simulink model "spindle_mileusnic"  (Simulink 7.0)
settings: Solver=ode23s  StartTime=0.0  StopTime=3  RelTol=1e-3
values from neighbouring files (symbols this model uses):
  a = [0.3; 0.3; 0.3]    [SetSpindleConstants.m]    (also in createRamp.m = velocity / tacc)
  beta0 = [0.0605; 0.0822; 0.0822]    [SetSpindleConstants.m]
  beta1 = [0.2592; nan; nan]    [SetSpindleConstants.m]
  beta2 = [nan; -0.0460; -0.0690]    [SetSpindleConstants.m]
  Cl = [1; 1; 1]    [SetSpindleConstants.m]
  Cs = [0.42; 0.42; 0.42]    [SetSpindleConstants.m]
  freq = [60; 60; 90]    [SetSpindleConstants.m]
  Gamma1 = [0.0289; nan; nan]    [SetSpindleConstants.m]
  Gamma2 = [nan; 0.0636; 0.0954]    [SetSpindleConstants.m]
  Gprim = [20000; 10000; 10000]    [SetSpindleConstants.m]
  Gsec = [nan; 7250; 7250]    [SetSpindleConstants.m]
  Kpr = [0.15; 0.15; 0.15]    [SetSpindleConstants.m]
  Ksr = [10.4549; 10.4649; 10.4649]    [SetSpindleConstants.m]
  L0pr = [0.76; 0.76; 0.76]    [SetSpindleConstants.m]
  L0sr = [0.04; 0.04; 0.04]    [SetSpindleConstants.m]
  Lnpr = [nan; 0.89; 0.89]    [SetSpindleConstants.m]
  Lnsr = [0.0423; 0.0423; 0.0423]    [SetSpindleConstants.m]
  Lsec = [nan; 0.04; 0.04]    [SetSpindleConstants.m]
  M = M/100    [SetSpindleConstants.m]
  p = [2; 2; 2]    [SetSpindleConstants.m]
  R = [0.46; 0.46; 0.46]    [SetSpindleConstants.m]
  S = (E >= TH)    [RampModel.m]    (also in SetSpindleConstants.m = 0.156; step3_plotResults.m = out{velIdx,ampIdx}.nrn.Sdetail)
  tau = [0.0149; 0.205; nan]    [SetSpindleConstants.m]
  X = [nan; 0.7; 0.7]    [SetSpindleConstants.m]
settings Model: Creator=Schuurmans  LastModifiedBy=jschuurmans1
settings DebuggingCC: SaveWithParameterizedLinksMsg=none  SignalResolutionControl=TryResolveAllWithWarning  SolverPrmCheckMsg=none
settings GRTTargetCC: TargetFcnLib=ansi_tfl_tmw.mat

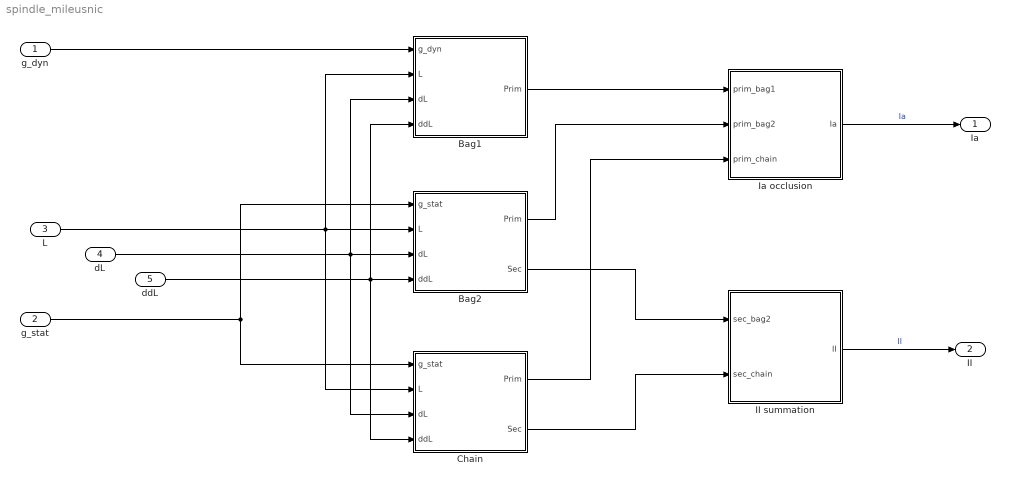
== system spindle_mileusnic ==
  g_dyn : Inport  OutDataType=sfix(16)  OutScaling=2^0
  g_stat : Inport  Port=2  OutDataType=sfix(16)  OutScaling=2^0
  L : Inport  Port=3  OutDataType=sfix(16)  OutScaling=2^0  Interpolate=off
  dL : Inport  Port=4  OutDataType=sfix(16)  OutScaling=2^0  Interpolate=off
  ddL : Inport  Port=5  OutDataType=sfix(16)  OutScaling=2^0  Interpolate=off
  Bag1 : Subsystem
  Bag2 : Subsystem
  Chain : Subsystem
  II summation : Subsystem
  Ia occlusion : Subsystem
  Ia : Outport  OutDataType=sfix(16)  OutScaling=2^0
  II : Outport  Port=2  OutDataType=sfix(16)  OutScaling=2^0
  wires:
  L/1 -> Bag2/2(L), Chain/2(L), Bag1/2(L)
  dL/1 -> Bag2/3(dL), Bag1/3(dL), Chain/3(dL)
  ddL/1 -> Bag2/4(ddL), Bag1/4(ddL), Chain/4(ddL)
  g_dyn/1 -> Bag1/1(g_dyn)
  g_stat/1 -> Bag2/1(g_stat), Chain/1(g_stat)
  Bag1/1(Prim) -> Ia occlusion/1(prim_bag1)
  Bag2/1(Prim) -> Ia occlusion/2(prim_bag2)
  Chain/1(Prim) -> Ia occlusion/3(prim_chain)
  Bag2/2(Sec) -> II summation/1(sec_bag2)
  Chain/2(Sec) -> II summation/2(sec_chain)
  II summation/1(II) -> II/1  "II"
  Ia occlusion/1(Ia) -> Ia/1  "Ia"

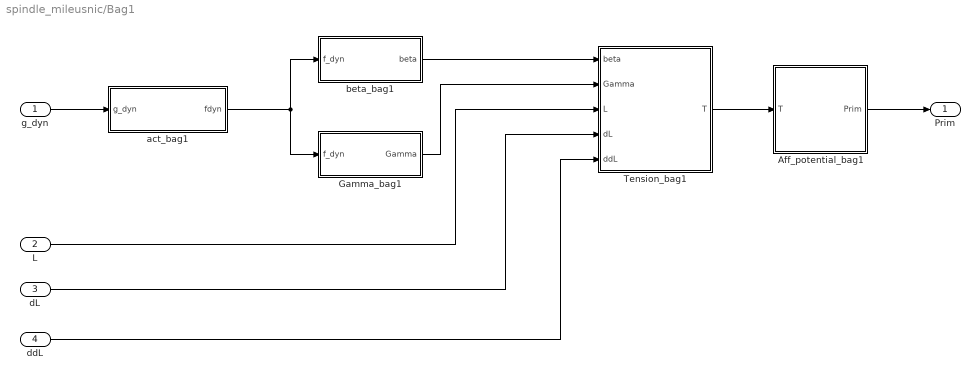
== system spindle_mileusnic/Bag1 ==
  g_dyn : Inport  OutDataType=sfix(16)  OutScaling=2^0
  L : Inport  Port=2  OutDataType=sfix(16)  OutScaling=2^0
  dL : Inport  Port=3  OutDataType=sfix(16)  OutScaling=2^0
  ddL : Inport  Port=4  OutDataType=sfix(16)  OutScaling=2^0
  Aff_potential_bag1 : Subsystem
  Gamma_bag1 : Subsystem
  Tension_bag1 : Subsystem
  act_bag1 : Subsystem
  beta_bag1 : Subsystem
  Prim : Outport  OutDataType=sfix(16)  OutScaling=2^0
  wires:
  act_bag1/1(fdyn) -> beta_bag1/1(f_dyn), Gamma_bag1/1(f_dyn)
  Gamma_bag1/1(Gamma) -> Tension_bag1/2(Gamma)
  Tension_bag1/1(T) -> Aff_potential_bag1/1(T)
  beta_bag1/1(beta) -> Tension_bag1/1(beta)
  g_dyn/1 -> act_bag1/1(g_dyn)
  L/1 -> Tension_bag1/3(L)
  dL/1 -> Tension_bag1/4(dL)
  ddL/1 -> Tension_bag1/5(ddL)
  Aff_potential_bag1/1(Prim) -> Prim/1

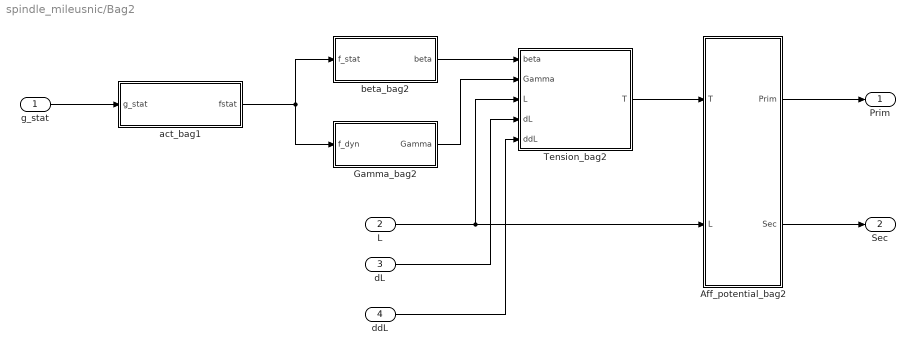
== system spindle_mileusnic/Bag2 ==
  g_stat : Inport  OutDataType=sfix(16)  OutScaling=2^0
  L : Inport  Port=2  OutDataType=sfix(16)  OutScaling=2^0
  dL : Inport  Port=3  OutDataType=sfix(16)  OutScaling=2^0
  ddL : Inport  Port=4  OutDataType=sfix(16)  OutScaling=2^0
  Aff_potential_bag2 : Subsystem
  Gamma_bag2 : Subsystem
  Tension_bag2 : Subsystem
  act_bag1 : Subsystem
  beta_bag2 : Subsystem
  Prim : Outport  OutDataType=sfix(16)  OutScaling=2^0
  Sec : Outport  Port=2  OutDataType=sfix(16)  OutScaling=2^0
  wires:
  g_stat/1 -> act_bag1/1(g_stat)
  beta_bag2/1(beta) -> Tension_bag2/1(beta)
  Gamma_bag2/1(Gamma) -> Tension_bag2/2(Gamma)
  act_bag1/1(fstat) -> beta_bag2/1(f_stat), Gamma_bag2/1(f_dyn)
  L/1 -> Tension_bag2/3(L), Aff_potential_bag2/2(L)
  dL/1 -> Tension_bag2/4(dL)
  ddL/1 -> Tension_bag2/5(ddL)
  Aff_potential_bag2/1(Prim) -> Prim/1
  Aff_potential_bag2/2(Sec) -> Sec/1
  Tension_bag2/1(T) -> Aff_potential_bag2/1(T)

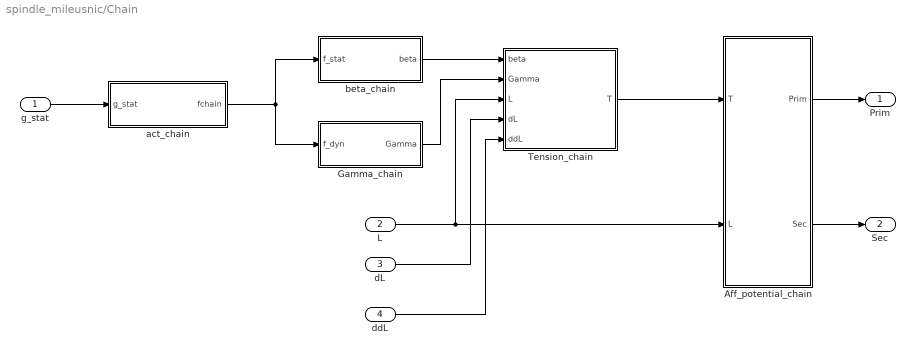
== system spindle_mileusnic/Chain ==
  g_stat : Inport  OutDataType=sfix(16)  OutScaling=2^0
  L : Inport  Port=2  OutDataType=sfix(16)  OutScaling=2^0
  dL : Inport  Port=3  OutDataType=sfix(16)  OutScaling=2^0
  ddL : Inport  Port=4  OutDataType=sfix(16)  OutScaling=2^0
  Aff_potential_chain : Subsystem
  Gamma_chain : Subsystem
  Tension_chain : Subsystem
  act_chain : Subsystem
  beta_chain : Subsystem
  Prim : Outport  OutDataType=sfix(16)  OutScaling=2^0
  Sec : Outport  Port=2  OutDataType=sfix(16)  OutScaling=2^0
  wires:
  beta_chain/1(beta) -> Tension_chain/1(beta)
  Gamma_chain/1(Gamma) -> Tension_chain/2(Gamma)
  act_chain/1(fchain) -> beta_chain/1(f_stat), Gamma_chain/1(f_dyn)
  g_stat/1 -> act_chain/1(g_stat)
  L/1 -> Tension_chain/3(L), Aff_potential_chain/2(L)
  dL/1 -> Tension_chain/4(dL)
  ddL/1 -> Tension_chain/5(ddL)
  Tension_chain/1(T) -> Aff_potential_chain/1(T)
  Aff_potential_chain/2(Sec) -> Sec/1
  Aff_potential_chain/1(Prim) -> Prim/1

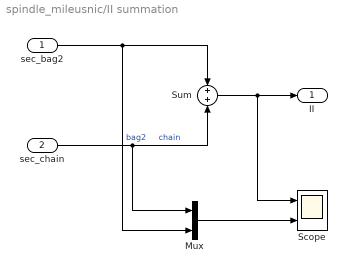
== system spindle_mileusnic/II summation ==
  sec_bag2 : Inport  OutDataType=sfix(16)  OutScaling=2^0
  sec_chain : Inport  Port=2  OutDataType=sfix(16)  OutScaling=2^0
  Mux : Mux  Inputs=2
  Scope : Scope  NumInputPorts=2
      settings: TickLabels=on  TimeRange=0.006999999999999673  YMin=0.00580385~-5  YMax=0.00580415~5  SaveName=ScopeData7
  Sum : Sum  OutDataType=sfix(16)  OutScaling=2^0
  II : Outport  OutDataType=sfix(16)  OutScaling=2^0
  wires:
  sec_bag2/1 -> Mux/2, Sum/1  "bag2"
  sec_chain/1 -> Sum/2, Mux/1  "chain"
  Sum/1 -> II/1, Scope/1
  Mux/1 -> Scope/2

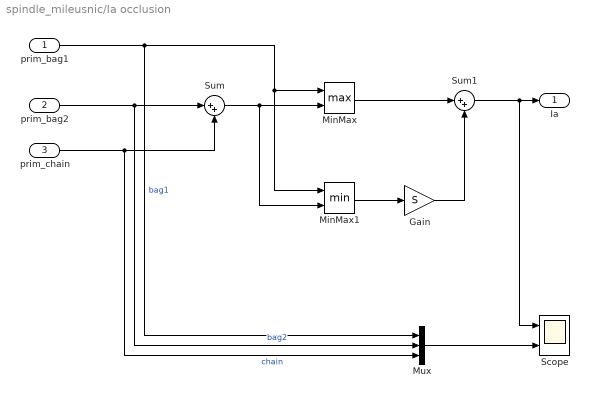
== system spindle_mileusnic/Ia occlusion ==
  prim_bag1 : Inport  OutDataType=sfix(16)  OutScaling=2^0
  prim_bag2 : Inport  Port=2  OutDataType=sfix(16)  OutScaling=2^0
  prim_chain : Inport  Port=3  OutDataType=sfix(16)  OutScaling=2^0
  Gain : Gain  Gain=S  ParameterDataType=sfix(16)  ParameterScaling=2^0  OutDataType=sfix(16)  OutScaling=2^0
  MinMax : MinMax  Function=max  Inputs=2  OutDataType=sfix(16)  OutScaling=2^0
  MinMax1 : MinMax  Inputs=2  OutDataType=sfix(16)  OutScaling=2^0
  Mux : Mux  Inputs=3
  Scope : Scope  NumInputPorts=2
      settings: TickLabels=on  TimeRange=0.006999999999999673  YMin=0.00580385~-5  YMax=0.00580415~5  SaveName=ScopeData5
  Sum : Sum  Inputs=|++  OutDataType=sfix(16)  OutScaling=2^0
  Sum1 : Sum  Inputs=|++  OutDataType=sfix(16)  OutScaling=2^0
  Ia : Outport  OutDataType=sfix(16)  OutScaling=2^0
  wires:
  prim_bag2/1 -> Sum/1, Mux/2  "bag2"
  prim_chain/1 -> Sum/2, Mux/3  "chain"
  prim_bag1/1 -> MinMax/1, MinMax1/1, Mux/1  "bag1"
  Sum/1 -> MinMax/2, MinMax1/2
  MinMax/1 -> Sum1/1
  MinMax1/1 -> Gain/1
  Gain/1 -> Sum1/2
  Sum1/1 -> Ia/1, Scope/1
  Mux/1 -> Scope/2

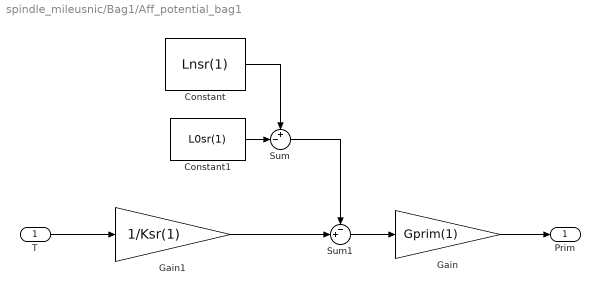
== system spindle_mileusnic/Bag1/Aff_potential_bag1 ==
  T : Inport  OutDataType=sfix(16)  OutScaling=2^0
  Constant : Constant  Value=Lnsr(1)  OutDataType=sfix(16)  OutScaling=2^0
  Constant1 : Constant  Value=L0sr(1)  OutDataType=sfix(16)  OutScaling=2^0
  Gain : Gain  Gain=Gprim(1)  ParameterDataType=sfix(16)  ParameterScaling=2^0  OutDataType=sfix(16)  OutScaling=2^0
  Gain1 : Gain  Gain=1/Ksr(1)  ParameterDataType=sfix(16)  ParameterScaling=2^0  OutDataType=sfix(16)  OutScaling=2^0
  Sum : Sum  Inputs=+-|  OutDataType=sfix(16)  OutScaling=2^0
  Sum1 : Sum  Inputs=-+|  OutDataType=sfix(16)  OutScaling=2^0
  Prim : Outport  OutDataType=sfix(16)  OutScaling=2^0
  wires:
  T/1 -> Gain1/1
  Constant1/1 -> Sum/2
  Constant/1 -> Sum/1
  Gain1/1 -> Sum1/2
  Sum/1 -> Sum1/1
  Sum1/1 -> Gain/1
  Gain/1 -> Prim/1

== system spindle_mileusnic/Bag1/Gamma_bag1 ==
  f_dyn : Inport  OutDataType=sfix(16)  OutScaling=2^0
  Gain : Gain  Gain=Gamma1(1)  ParameterDataType=sfix(16)  ParameterScaling=2^0  OutDataType=sfix(16)  OutScaling=2^0
  Gamma : Outport  OutDataType=sfix(16)  OutScaling=2^0
  wires:
  f_dyn/1 -> Gain/1
  Gain/1 -> Gamma/1

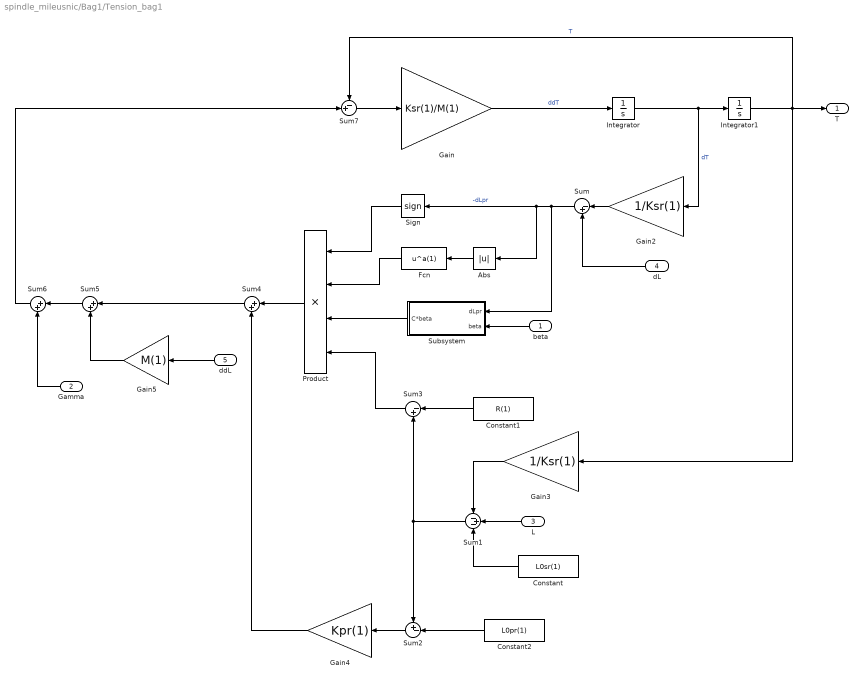
== system spindle_mileusnic/Bag1/Tension_bag1 ==
  beta : Inport  Orientation=left  OutDataType=sfix(16)  OutScaling=2^0
  Gamma : Inport  Orientation=left  Port=2  OutDataType=sfix(16)  OutScaling=2^0
  L : Inport  Orientation=left  Port=3  OutDataType=sfix(16)  OutScaling=2^0
  dL : Inport  Orientation=left  Port=4  OutDataType=sfix(16)  OutScaling=2^0
  ddL : Inport  Orientation=left  Port=5  OutDataType=sfix(16)  OutScaling=2^0
  Abs : Abs  Orientation=left  ZeroCross=off
  Constant : Constant  Orientation=left  Value=L0sr(1)  OutDataType=sfix(16)  OutScaling=2^0
  Constant1 : Constant  Orientation=left  Value=R(1)  OutDataType=sfix(16)  OutScaling=2^0
  Constant2 : Constant  Orientation=left  Value=L0pr(1)  OutDataType=sfix(16)  OutScaling=2^0
  Fcn : Fcn  Orientation=left  Expr=u^a(1)
  Gain : Gain  Gain=Ksr(1)/M(1)  ParameterDataType=sfix(16)  ParameterScaling=2^0  OutDataType=sfix(16)  OutScaling=2^0
  Gain2 : Gain  Orientation=left  Gain=1/Ksr(1)  ParameterDataType=sfix(16)  ParameterScaling=2^0  OutDataType=sfix(16)  OutScaling=2^0
  Gain3 : Gain  Orientation=left  Gain=1/Ksr(1)  ParameterDataType=sfix(16)  ParameterScaling=2^0  OutDataType=sfix(16)  OutScaling=2^0
  Gain4 : Gain  Orientation=left  Gain=Kpr(1)  ParameterDataType=sfix(16)  ParameterScaling=2^0  OutDataType=sfix(16)  OutScaling=2^0
  Gain5 : Gain  Orientation=left  Gain=M(1)  ParameterDataType=sfix(16)  ParameterScaling=2^0  OutDataType=sfix(16)  OutScaling=2^0
  Integrator : Integrator
  Integrator1 : Integrator
  Product : Product  Orientation=left  Inputs=4  OutDataType=sfix(16)  OutScaling=2^0  RndMeth=Zero
  Sign : Signum  Orientation=left  ZeroCross=off
  Subsystem : Subsystem  Orientation=left
  Sum : Sum  Orientation=left  Inputs=|-+  OutDataType=sfix(16)  OutScaling=2^0
  Sum1 : Sum  Orientation=left  Inputs=-+-  OutDataType=sfix(16)  OutScaling=2^0
  Sum2 : Sum  Orientation=left  Inputs=+-|  OutDataType=sfix(16)  OutScaling=2^0
  Sum3 : Sum  Orientation=left  Inputs=|-+  OutDataType=sfix(16)  OutScaling=2^0
  Sum4 : Sum  Orientation=left  Inputs=|++  OutDataType=sfix(16)  OutScaling=2^0
  Sum5 : Sum  Orientation=left  Inputs=|++  OutDataType=sfix(16)  OutScaling=2^0
  Sum6 : Sum  Orientation=left  Inputs=|++  OutDataType=sfix(16)  OutScaling=2^0
  Sum7 : Sum  Inputs=-+|  OutDataType=sfix(16)  OutScaling=2^0
  T : Outport  OutDataType=sfix(16)  OutScaling=2^0
  wires:
  Integrator/1 -> Integrator1/1, Gain2/1  "dT"
  Integrator1/1 -> Gain3/1, Sum7/1, T/1  "T"
  Gain/1 -> Integrator/1  "ddT"
  dL/1 -> Sum/2
  Gain2/1 -> Sum/1
  Sum/1 -> Sign/1, Abs/1, Subsystem/1(dLpr)  "-dLpr"
  Abs/1 -> Fcn/1
  Sign/1 -> Product/1
  Fcn/1 -> Product/2
  Sum3/1 -> Product/4
  L/1 -> Sum1/2
  Gain3/1 -> Sum1/1
  Constant/1 -> Sum1/3
  Sum1/1 -> Sum3/2, Sum2/1
  Constant1/1 -> Sum3/1
  Constant2/1 -> Sum2/2
  Sum2/1 -> Gain4/1
  ddL/1 -> Gain5/1
  Product/1 -> Sum4/1
  Gain4/1 -> Sum4/2
  Sum4/1 -> Sum5/1
  Gain5/1 -> Sum5/2
  Sum5/1 -> Sum6/1
  Gamma/1 -> Sum6/2
  Sum6/1 -> Sum7/2
  Sum7/1 -> Gain/1
  beta/1 -> Subsystem/2(beta)
  Subsystem/1(C*beta) -> Product/3

== system spindle_mileusnic/Bag1/act_bag1 ==
  g_dyn : Inport  OutDataType=sfix(16)  OutScaling=2^0
  Fcn : Fcn  Expr=u^p(1) / (u^p(1) + freq(1)^p(1))
  Gain : Gain  Gain=1/tau(1)  ParameterDataType=sfix(16)  ParameterScaling=2^0  OutDataType=sfix(16)  OutScaling=2^0
  Integrator : Integrator
  Sum : Sum  Inputs=|+-  OutDataType=sfix(16)  OutScaling=2^0
  fdyn : Outport  OutDataType=sfix(16)  OutScaling=2^0
  wires:
  Integrator/1 -> Sum/2, fdyn/1
  g_dyn/1 -> Fcn/1
  Fcn/1 -> Sum/1
  Gain/1 -> Integrator/1
  Sum/1 -> Gain/1

== system spindle_mileusnic/Bag1/beta_bag1 ==
  f_dyn : Inport  OutDataType=sfix(16)  OutScaling=2^0
  Gain : Gain  Gain=beta1(1)  ParameterDataType=sfix(16)  ParameterScaling=2^0  OutDataType=sfix(16)  OutScaling=2^0
  Sum : Sum  Inputs=|++  OutDataType=sfix(16)  OutScaling=2^0
  beta0 : Constant  Value=beta0(1)  OutDataType=sfix(16)  OutScaling=2^0
  beta : Outport  OutDataType=sfix(16)  OutScaling=2^0
  wires:
  f_dyn/1 -> Gain/1
  Gain/1 -> Sum/1
  beta0/1 -> Sum/2
  Sum/1 -> beta/1

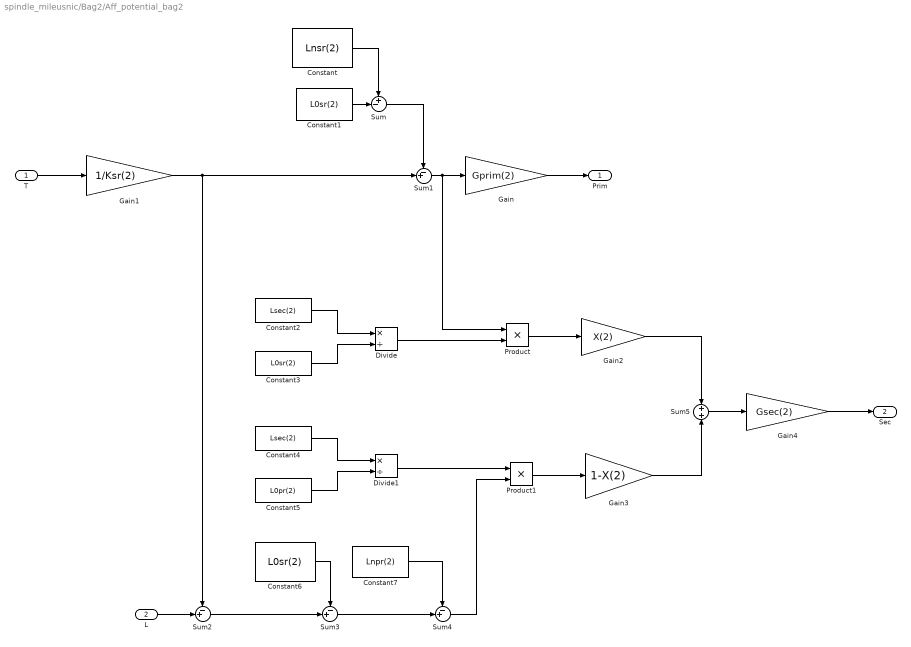
== system spindle_mileusnic/Bag2/Aff_potential_bag2 ==
  T : Inport  OutDataType=sfix(16)  OutScaling=2^0
  L : Inport  Port=2  OutDataType=sfix(16)  OutScaling=2^0
  Constant : Constant  Value=Lnsr(2)  OutDataType=sfix(16)  OutScaling=2^0
  Constant1 : Constant  Value=L0sr(2)  OutDataType=sfix(16)  OutScaling=2^0
  Constant2 : Constant  Value=Lsec(2)  OutDataType=sfix(16)  OutScaling=2^0
  Constant3 : Constant  Value=L0sr(2)  OutDataType=sfix(16)  OutScaling=2^0
  Constant4 : Constant  Value=Lsec(2)  OutDataType=sfix(16)  OutScaling=2^0
  Constant5 : Constant  Value=L0pr(2)  OutDataType=sfix(16)  OutScaling=2^0
  Constant6 : Constant  Value=L0sr(2)  OutDataType=sfix(16)  OutScaling=2^0
  Constant7 : Constant  Value=Lnpr(2)  OutDataType=sfix(16)  OutScaling=2^0
  Divide : Product  Inputs=*/  OutDataType=sfix(16)  OutScaling=2^-10
  Divide1 : Product  Inputs=*/  OutDataType=sfix(16)  OutScaling=2^-10
  Gain : Gain  Gain=Gprim(2)  ParameterDataType=sfix(16)  ParameterScaling=2^0  OutDataType=sfix(16)  OutScaling=2^0
  Gain1 : Gain  Gain=1/Ksr(2)  ParameterDataType=sfix(16)  ParameterScaling=2^0  OutDataType=sfix(16)  OutScaling=2^0
  Gain2 : Gain  Gain=X(2)  ParameterDataType=sfix(16)  ParameterScaling=2^0  OutDataType=sfix(16)  OutScaling=2^0
  Gain3 : Gain  Gain=1-X(2)  ParameterDataType=sfix(16)  ParameterScaling=2^0  OutDataType=sfix(16)  OutScaling=2^0
  Gain4 : Gain  Gain=Gsec(2)  ParameterDataType=sfix(16)  ParameterScaling=2^0  OutDataType=sfix(16)  OutScaling=2^0
  Product : Product  OutDataType=sfix(16)  OutScaling=2^0  RndMeth=Zero
  Product1 : Product  OutDataType=sfix(16)  OutScaling=2^0  RndMeth=Zero
  Sum : Sum  Inputs=+-|  OutDataType=sfix(16)  OutScaling=2^0
  Sum{1..4} (4 alike) : Sum  Inputs=-+|  OutDataType=sfix(16)  OutScaling=2^0
  Sum5 : Sum  Inputs=+|+  OutDataType=sfix(16)  OutScaling=2^0
  Prim : Outport  OutDataType=sfix(16)  OutScaling=2^0
  Sec : Outport  Port=2  OutDataType=sfix(16)  OutScaling=2^0
  wires:
  T/1 -> Gain1/1
  Constant1/1 -> Sum/2
  Constant/1 -> Sum/1
  Gain1/1 -> Sum1/2, Sum2/1
  Sum/1 -> Sum1/1
  Sum1/1 -> Gain/1, Product/1
  Gain/1 -> Prim/1
  Constant2/1 -> Divide/1
  Constant3/1 -> Divide/2
  Divide/1 -> Product/2
  Product/1 -> Gain2/1
  Constant4/1 -> Divide1/1
  Constant5/1 -> Divide1/2
  L/1 -> Sum2/2
  Sum2/1 -> Sum3/2
  Constant6/1 -> Sum3/1
  Sum3/1 -> Sum4/2
  Constant7/1 -> Sum4/1
  Divide1/1 -> Product1/1
  Sum4/1 -> Product1/2
  Product1/1 -> Gain3/1
  Gain2/1 -> Sum5/1
  Gain3/1 -> Sum5/2
  Sum5/1 -> Gain4/1
  Gain4/1 -> Sec/1

== system spindle_mileusnic/Bag2/Gamma_bag2 ==
  f_dyn : Inport  OutDataType=sfix(16)  OutScaling=2^0
  Gain : Gain  Gain=Gamma2(2)  ParameterDataType=sfix(16)  ParameterScaling=2^0  OutDataType=sfix(16)  OutScaling=2^0
  Gamma : Outport  OutDataType=sfix(16)  OutScaling=2^0
  wires:
  f_dyn/1 -> Gain/1
  Gain/1 -> Gamma/1

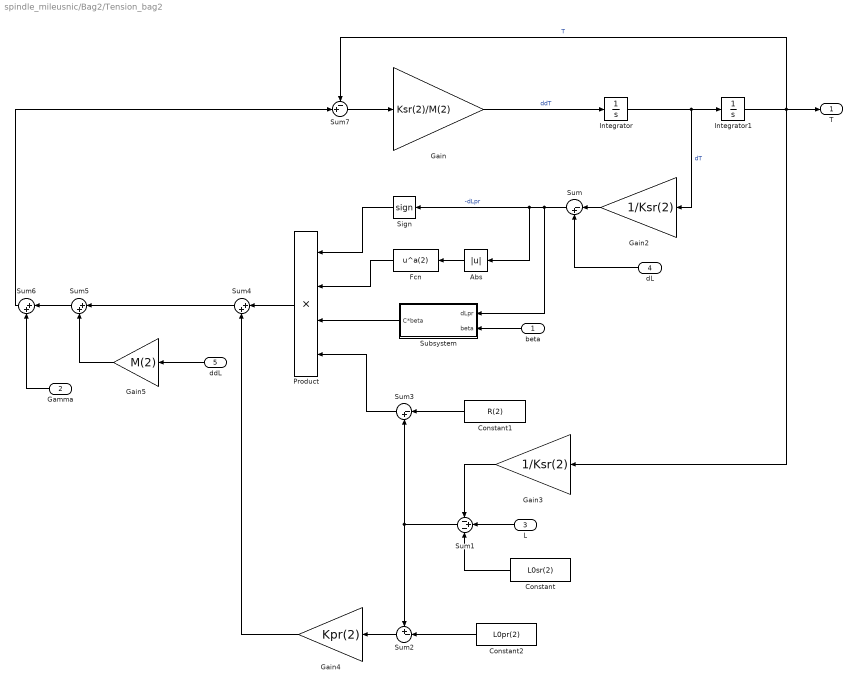
== system spindle_mileusnic/Bag2/Tension_bag2 ==
  beta : Inport  Orientation=left  OutDataType=sfix(16)  OutScaling=2^0
  Gamma : Inport  Orientation=left  Port=2  OutDataType=sfix(16)  OutScaling=2^0
  L : Inport  Orientation=left  Port=3  OutDataType=sfix(16)  OutScaling=2^0
  dL : Inport  Orientation=left  Port=4  OutDataType=sfix(16)  OutScaling=2^0
  ddL : Inport  Orientation=left  Port=5  OutDataType=sfix(16)  OutScaling=2^0
  Abs : Abs  Orientation=left  ZeroCross=off
  Constant : Constant  Orientation=left  Value=L0sr(2)  OutDataType=sfix(16)  OutScaling=2^0
  Constant1 : Constant  Orientation=left  Value=R(2)  OutDataType=sfix(16)  OutScaling=2^0
  Constant2 : Constant  Orientation=left  Value=L0pr(2)  OutDataType=sfix(16)  OutScaling=2^0
  Fcn : Fcn  Orientation=left  Expr=u^a(2)
  Gain : Gain  Gain=Ksr(2)/M(2)  ParameterDataType=sfix(16)  ParameterScaling=2^0  OutDataType=sfix(16)  OutScaling=2^0
  Gain2 : Gain  Orientation=left  Gain=1/Ksr(2)  ParameterDataType=sfix(16)  ParameterScaling=2^0  OutDataType=sfix(16)  OutScaling=2^0
  Gain3 : Gain  Orientation=left  Gain=1/Ksr(2)  ParameterDataType=sfix(16)  ParameterScaling=2^0  OutDataType=sfix(16)  OutScaling=2^0
  Gain4 : Gain  Orientation=left  Gain=Kpr(2)  ParameterDataType=sfix(16)  ParameterScaling=2^0  OutDataType=sfix(16)  OutScaling=2^0
  Gain5 : Gain  Orientation=left  Gain=M(2)  ParameterDataType=sfix(16)  ParameterScaling=2^0  OutDataType=sfix(16)  OutScaling=2^0
  Integrator : Integrator
  Integrator1 : Integrator
  Product : Product  Orientation=left  Inputs=4  OutDataType=sfix(16)  OutScaling=2^0  RndMeth=Zero
  Sign : Signum  Orientation=left  ZeroCross=off
  Subsystem : Subsystem  Orientation=left
  Sum : Sum  Orientation=left  Inputs=|-+  OutDataType=sfix(16)  OutScaling=2^0
  Sum1 : Sum  Orientation=left  Inputs=-+-  OutDataType=sfix(16)  OutScaling=2^0
  Sum2 : Sum  Orientation=left  Inputs=+-|  OutDataType=sfix(16)  OutScaling=2^0
  Sum3 : Sum  Orientation=left  Inputs=|-+  OutDataType=sfix(16)  OutScaling=2^0
  Sum4 : Sum  Orientation=left  Inputs=|++  OutDataType=sfix(16)  OutScaling=2^0
  Sum5 : Sum  Orientation=left  Inputs=|++  OutDataType=sfix(16)  OutScaling=2^0
  Sum6 : Sum  Orientation=left  Inputs=|++  OutDataType=sfix(16)  OutScaling=2^0
  Sum7 : Sum  Inputs=-+|  OutDataType=sfix(16)  OutScaling=2^0
  T : Outport  OutDataType=sfix(16)  OutScaling=2^0
  wires:
  Integrator/1 -> Integrator1/1, Gain2/1  "dT"
  Integrator1/1 -> Gain3/1, Sum7/1, T/1  "T"
  Gain/1 -> Integrator/1  "ddT"
  dL/1 -> Sum/2
  Gain2/1 -> Sum/1
  Sum/1 -> Sign/1, Abs/1, Subsystem/1(dLpr)  "-dLpr"
  Abs/1 -> Fcn/1
  Sign/1 -> Product/1
  Fcn/1 -> Product/2
  Sum3/1 -> Product/4
  L/1 -> Sum1/2
  Gain3/1 -> Sum1/1
  Constant/1 -> Sum1/3
  Sum1/1 -> Sum3/2, Sum2/1
  Constant1/1 -> Sum3/1
  Constant2/1 -> Sum2/2
  Sum2/1 -> Gain4/1
  ddL/1 -> Gain5/1
  Product/1 -> Sum4/1
  Gain4/1 -> Sum4/2
  Sum4/1 -> Sum5/1
  Gain5/1 -> Sum5/2
  Sum5/1 -> Sum6/1
  Gamma/1 -> Sum6/2
  Sum6/1 -> Sum7/2
  Sum7/1 -> Gain/1
  beta/1 -> Subsystem/2(beta)
  Subsystem/1(C*beta) -> Product/3

== system spindle_mileusnic/Bag2/act_bag1 ==
  g_stat : Inport  OutDataType=sfix(16)  OutScaling=2^0
  Fcn : Fcn  Expr=u^p(2) / (u^p(2) + freq(2)^p(2))
  Gain : Gain  Gain=1/tau(2)  ParameterDataType=sfix(16)  ParameterScaling=2^0  OutDataType=sfix(16)  OutScaling=2^0
  Integrator : Integrator
  Sum : Sum  Inputs=|+-  OutDataType=sfix(16)  OutScaling=2^0
  fstat : Outport  OutDataType=sfix(16)  OutScaling=2^0
  wires:
  Integrator/1 -> fstat/1, Sum/2
  g_stat/1 -> Fcn/1
  Fcn/1 -> Sum/1
  Gain/1 -> Integrator/1
  Sum/1 -> Gain/1

== system spindle_mileusnic/Bag2/beta_bag2 ==
  f_stat : Inport  OutDataType=sfix(16)  OutScaling=2^0
  Gain : Gain  Gain=beta2(2)  ParameterDataType=sfix(16)  ParameterScaling=2^0  OutDataType=sfix(16)  OutScaling=2^0
  Sum : Sum  Inputs=|++  OutDataType=sfix(16)  OutScaling=2^0
  beta0 : Constant  Value=beta0(2)  OutDataType=sfix(16)  OutScaling=2^0
  beta : Outport  OutDataType=sfix(16)  OutScaling=2^0
  wires:
  f_stat/1 -> Gain/1
  Gain/1 -> Sum/1
  beta0/1 -> Sum/2
  Sum/1 -> beta/1

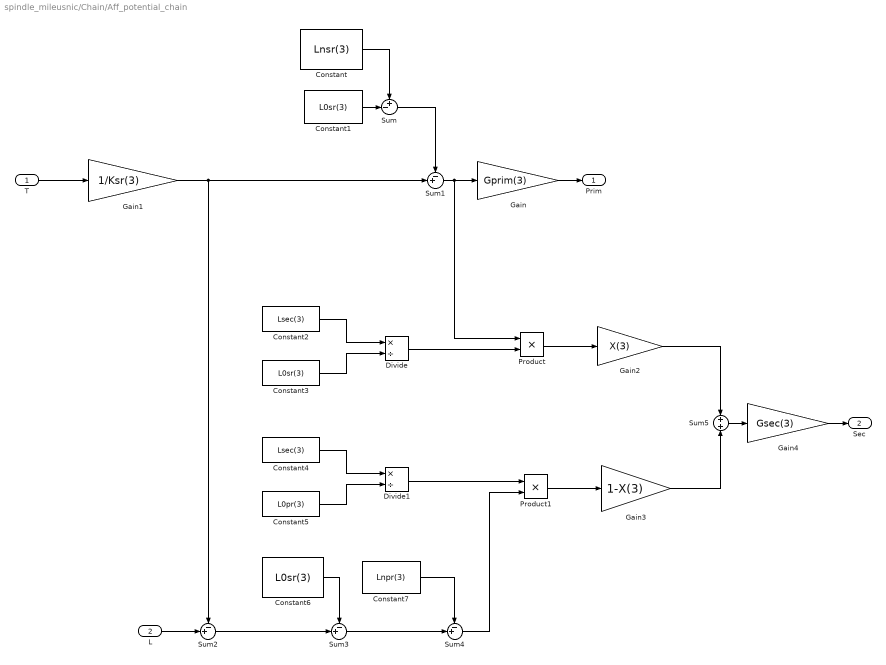
== system spindle_mileusnic/Chain/Aff_potential_chain ==
  T : Inport  OutDataType=sfix(16)  OutScaling=2^0
  L : Inport  Port=2  OutDataType=sfix(16)  OutScaling=2^0
  Constant : Constant  Value=Lnsr(3)  OutDataType=sfix(16)  OutScaling=2^0
  Constant1 : Constant  Value=L0sr(3)  OutDataType=sfix(16)  OutScaling=2^0
  Constant2 : Constant  Value=Lsec(3)  OutDataType=sfix(16)  OutScaling=2^0
  Constant3 : Constant  Value=L0sr(3)  OutDataType=sfix(16)  OutScaling=2^0
  Constant4 : Constant  Value=Lsec(3)  OutDataType=sfix(16)  OutScaling=2^0
  Constant5 : Constant  Value=L0pr(3)  OutDataType=sfix(16)  OutScaling=2^0
  Constant6 : Constant  Value=L0sr(3)  OutDataType=sfix(16)  OutScaling=2^0
  Constant7 : Constant  Value=Lnpr(3)  OutDataType=sfix(16)  OutScaling=2^0
  Divide : Product  Inputs=*/  OutDataType=sfix(16)  OutScaling=2^-10
  Divide1 : Product  Inputs=*/  OutDataType=sfix(16)  OutScaling=2^-10
  Gain : Gain  Gain=Gprim(3)  ParameterDataType=sfix(16)  ParameterScaling=2^0  OutDataType=sfix(16)  OutScaling=2^0
  Gain1 : Gain  Gain=1/Ksr(3)  ParameterDataType=sfix(16)  ParameterScaling=2^0  OutDataType=sfix(16)  OutScaling=2^0
  Gain2 : Gain  Gain=X(3)  ParameterDataType=sfix(16)  ParameterScaling=2^0  OutDataType=sfix(16)  OutScaling=2^0
  Gain3 : Gain  Gain=1-X(3)  ParameterDataType=sfix(16)  ParameterScaling=2^0  OutDataType=sfix(16)  OutScaling=2^0
  Gain4 : Gain  Gain=Gsec(3)  ParameterDataType=sfix(16)  ParameterScaling=2^0  OutDataType=sfix(16)  OutScaling=2^0
  Product : Product  OutDataType=sfix(16)  OutScaling=2^0  RndMeth=Zero
  Product1 : Product  OutDataType=sfix(16)  OutScaling=2^0  RndMeth=Zero
  Sum : Sum  Inputs=+-|  OutDataType=sfix(16)  OutScaling=2^0
  Sum{1..4} (4 alike) : Sum  Inputs=-+|  OutDataType=sfix(16)  OutScaling=2^0
  Sum5 : Sum  Inputs=+|+  OutDataType=sfix(16)  OutScaling=2^0
  Prim : Outport  OutDataType=sfix(16)  OutScaling=2^0
  Sec : Outport  Port=2  OutDataType=sfix(16)  OutScaling=2^0
  wires:
  T/1 -> Gain1/1
  Constant1/1 -> Sum/2
  Constant/1 -> Sum/1
  Gain1/1 -> Sum1/2, Sum2/1
  Sum/1 -> Sum1/1
  Sum1/1 -> Gain/1, Product/1
  Gain/1 -> Prim/1
  Constant2/1 -> Divide/1
  Constant3/1 -> Divide/2
  Divide/1 -> Product/2
  Product/1 -> Gain2/1
  Constant4/1 -> Divide1/1
  Constant5/1 -> Divide1/2
  L/1 -> Sum2/2
  Sum2/1 -> Sum3/2
  Constant6/1 -> Sum3/1
  Sum3/1 -> Sum4/2
  Constant7/1 -> Sum4/1
  Divide1/1 -> Product1/1
  Sum4/1 -> Product1/2
  Product1/1 -> Gain3/1
  Gain2/1 -> Sum5/1
  Gain3/1 -> Sum5/2
  Sum5/1 -> Gain4/1
  Gain4/1 -> Sec/1

== system spindle_mileusnic/Chain/Gamma_chain ==
  f_dyn : Inport  OutDataType=sfix(16)  OutScaling=2^0
  Gain : Gain  Gain=Gamma2(3)  ParameterDataType=sfix(16)  ParameterScaling=2^0  OutDataType=sfix(16)  OutScaling=2^0
  Gamma : Outport  OutDataType=sfix(16)  OutScaling=2^0
  wires:
  f_dyn/1 -> Gain/1
  Gain/1 -> Gamma/1

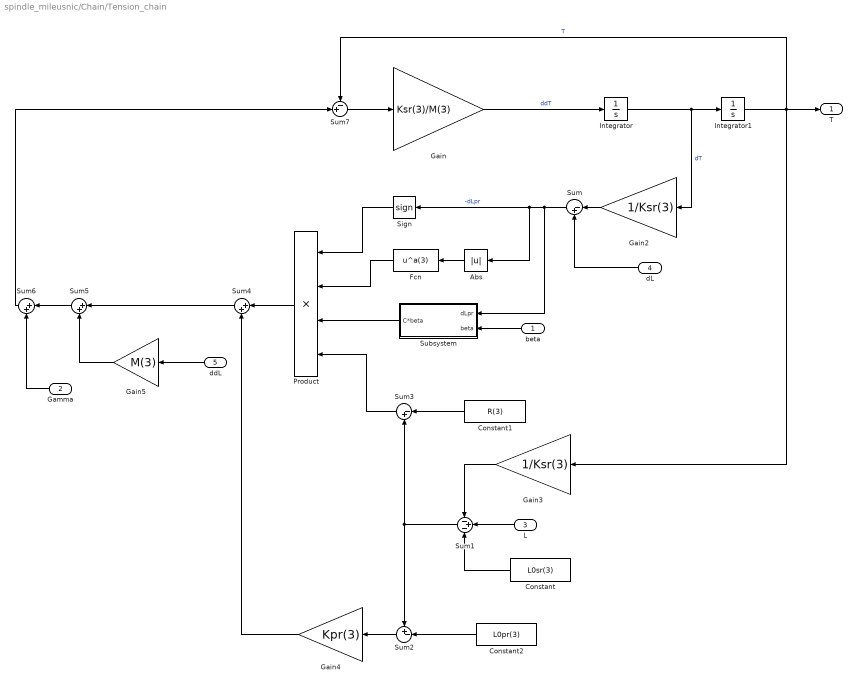
== system spindle_mileusnic/Chain/Tension_chain ==
  beta : Inport  Orientation=left  OutDataType=sfix(16)  OutScaling=2^0
  Gamma : Inport  Orientation=left  Port=2  OutDataType=sfix(16)  OutScaling=2^0
  L : Inport  Orientation=left  Port=3  OutDataType=sfix(16)  OutScaling=2^0
  dL : Inport  Orientation=left  Port=4  OutDataType=sfix(16)  OutScaling=2^0
  ddL : Inport  Orientation=left  Port=5  OutDataType=sfix(16)  OutScaling=2^0
  Abs : Abs  Orientation=left  ZeroCross=off
  Constant : Constant  Orientation=left  Value=L0sr(3)  OutDataType=sfix(16)  OutScaling=2^0
  Constant1 : Constant  Orientation=left  Value=R(3)  OutDataType=sfix(16)  OutScaling=2^0
  Constant2 : Constant  Orientation=left  Value=L0pr(3)  OutDataType=sfix(16)  OutScaling=2^0
  Fcn : Fcn  Orientation=left  Expr=u^a(3)
  Gain : Gain  Gain=Ksr(3)/M(3)  ParameterDataType=sfix(16)  ParameterScaling=2^0  OutDataType=sfix(16)  OutScaling=2^0
  Gain2 : Gain  Orientation=left  Gain=1/Ksr(3)  ParameterDataType=sfix(16)  ParameterScaling=2^0  OutDataType=sfix(16)  OutScaling=2^0
  Gain3 : Gain  Orientation=left  Gain=1/Ksr(3)  ParameterDataType=sfix(16)  ParameterScaling=2^0  OutDataType=sfix(16)  OutScaling=2^0
  Gain4 : Gain  Orientation=left  Gain=Kpr(3)  ParameterDataType=sfix(16)  ParameterScaling=2^0  OutDataType=sfix(16)  OutScaling=2^0
  Gain5 : Gain  Orientation=left  Gain=M(3)  ParameterDataType=sfix(16)  ParameterScaling=2^0  OutDataType=sfix(16)  OutScaling=2^0
  Integrator : Integrator
  Integrator1 : Integrator
  Product : Product  Orientation=left  Inputs=4  OutDataType=sfix(16)  OutScaling=2^0  RndMeth=Zero
  Sign : Signum  Orientation=left  ZeroCross=off
  Subsystem : Subsystem  Orientation=left
  Sum : Sum  Orientation=left  Inputs=|-+  OutDataType=sfix(16)  OutScaling=2^0
  Sum1 : Sum  Orientation=left  Inputs=-+-  OutDataType=sfix(16)  OutScaling=2^0
  Sum2 : Sum  Orientation=left  Inputs=+-|  OutDataType=sfix(16)  OutScaling=2^0
  Sum3 : Sum  Orientation=left  Inputs=|-+  OutDataType=sfix(16)  OutScaling=2^0
  Sum4 : Sum  Orientation=left  Inputs=|++  OutDataType=sfix(16)  OutScaling=2^0
  Sum5 : Sum  Orientation=left  Inputs=|++  OutDataType=sfix(16)  OutScaling=2^0
  Sum6 : Sum  Orientation=left  Inputs=|++  OutDataType=sfix(16)  OutScaling=2^0
  Sum7 : Sum  Inputs=-+|  OutDataType=sfix(16)  OutScaling=2^0
  T : Outport  OutDataType=sfix(16)  OutScaling=2^0
  wires:
  Integrator/1 -> Integrator1/1, Gain2/1  "dT"
  Integrator1/1 -> Gain3/1, Sum7/1, T/1  "T"
  Gain/1 -> Integrator/1  "ddT"
  dL/1 -> Sum/2
  Gain2/1 -> Sum/1
  Sum/1 -> Sign/1, Abs/1, Subsystem/1(dLpr)  "-dLpr"
  Abs/1 -> Fcn/1
  Sign/1 -> Product/1
  Fcn/1 -> Product/2
  Sum3/1 -> Product/4
  L/1 -> Sum1/2
  Gain3/1 -> Sum1/1
  Constant/1 -> Sum1/3
  Sum1/1 -> Sum3/2, Sum2/1
  Constant1/1 -> Sum3/1
  Constant2/1 -> Sum2/2
  Sum2/1 -> Gain4/1
  ddL/1 -> Gain5/1
  Product/1 -> Sum4/1
  Gain4/1 -> Sum4/2
  Sum4/1 -> Sum5/1
  Gain5/1 -> Sum5/2
  Sum5/1 -> Sum6/1
  Gamma/1 -> Sum6/2
  Sum6/1 -> Sum7/2
  Sum7/1 -> Gain/1
  beta/1 -> Subsystem/2(beta)
  Subsystem/1(C*beta) -> Product/3

== system spindle_mileusnic/Chain/act_chain ==
  g_stat : Inport  OutDataType=sfix(16)  OutScaling=2^0
  Fcn : Fcn  Expr=u^p(3) / (u^p(3) + freq(3)^p(3))
  fchain : Outport  OutDataType=sfix(16)  OutScaling=2^0
  wires:
  g_stat/1 -> Fcn/1
  Fcn/1 -> fchain/1

== system spindle_mileusnic/Chain/beta_chain ==
  f_stat : Inport  OutDataType=sfix(16)  OutScaling=2^0
  Gain : Gain  Gain=beta2(3)  ParameterDataType=sfix(16)  ParameterScaling=2^0  OutDataType=sfix(16)  OutScaling=2^0
  Sum : Sum  Inputs=|++  OutDataType=sfix(16)  OutScaling=2^0
  beta0 : Constant  Value=beta0(3)  OutDataType=sfix(16)  OutScaling=2^0
  beta : Outport  OutDataType=sfix(16)  OutScaling=2^0
  wires:
  f_stat/1 -> Gain/1
  Gain/1 -> Sum/1
  beta0/1 -> Sum/2
  Sum/1 -> beta/1

== system spindle_mileusnic/Bag1/Tension_bag1/Subsystem ==
  dLpr : Inport  OutDataType=sfix(16)  OutScaling=2^0
  beta : Inport  Port=2  OutDataType=sfix(16)  OutScaling=2^0
  Gain1 : Gain  Gain=Cl(1)  ParameterDataType=sfix(16)  ParameterScaling=2^0  OutDataType=sfix(16)  OutScaling=2^0
  Gain2 : Gain  Gain=Cs(1)  ParameterDataType=sfix(16)  ParameterScaling=2^0  OutDataType=sfix(16)  OutScaling=2^0
  Switch : Switch  ZeroCross=off
  C*beta : Outport  OutDataType=sfix(16)  OutScaling=2^0
  wires:
  Gain1/1 -> Switch/1
  Gain2/1 -> Switch/3
  Switch/1 -> C*beta/1
  beta/1 -> Gain1/1, Gain2/1
  dLpr/1 -> Switch/2

== system spindle_mileusnic/Bag2/Tension_bag2/Subsystem ==
  dLpr : Inport  OutDataType=sfix(16)  OutScaling=2^0
  beta : Inport  Port=2  OutDataType=sfix(16)  OutScaling=2^0
  Gain1 : Gain  Gain=Cl(2)  ParameterDataType=sfix(16)  ParameterScaling=2^0  OutDataType=sfix(16)  OutScaling=2^0
  Gain2 : Gain  Gain=Cs(2)  ParameterDataType=sfix(16)  ParameterScaling=2^0  OutDataType=sfix(16)  OutScaling=2^0
  Switch : Switch  ZeroCross=off
  C*beta : Outport  OutDataType=sfix(16)  OutScaling=2^0
  wires:
  Gain1/1 -> Switch/1
  Gain2/1 -> Switch/3
  Switch/1 -> C*beta/1
  beta/1 -> Gain1/1, Gain2/1
  dLpr/1 -> Switch/2

== system spindle_mileusnic/Chain/Tension_chain/Subsystem ==
  dLpr : Inport  OutDataType=sfix(16)  OutScaling=2^0
  beta : Inport  Port=2  OutDataType=sfix(16)  OutScaling=2^0
  Gain1 : Gain  Gain=Cl(3)  ParameterDataType=sfix(16)  ParameterScaling=2^0  OutDataType=sfix(16)  OutScaling=2^0
  Gain2 : Gain  Gain=Cs(3)  ParameterDataType=sfix(16)  ParameterScaling=2^0  OutDataType=sfix(16)  OutScaling=2^0
  Switch : Switch  ZeroCross=off
  C*beta : Outport  OutDataType=sfix(16)  OutScaling=2^0
  wires:
  Gain1/1 -> Switch/1
  Gain2/1 -> Switch/3
  Switch/1 -> C*beta/1
  beta/1 -> Gain1/1, Gain2/1
  dLpr/1 -> Switch/2
